simulink model "graphical_function4_2018a"  (R2018a)
settings: Solver=FixedStepDiscrete  StartTime=0.0  StopTime=1  FixedStep=0.1  RelTol=1e-3  EnableMultiTasking=on
settings Model: Creator=bzhan  LastModifiedBy=86188
settings SolverCC: AutoInsertRateTranBlk=on
settings DataIOCC: LimitDataPoints=on  ReturnWorkspaceOutputs=on
settings OptimizationCC: LifeSpan=inf
settings DebuggingCC: AllowSymbolicDim=off  SFUnexpectedBacktrackingDiag=warning  SFNoUnconditionalDefaultTransitionDiag=warning  SFExecutionAtInitializationDiag=none
settings CodeAppCC: StateflowObjectComments=on
settings GRTTargetCC: TargetLangStandard=C89/C90 (ANSI)
settings ConfigComp: CovMetricSettings=dw  CovHtmlReporting=on  CovSaveCumulativeToWorkspaceVar=on  CovSaveSingleToWorkspaceVar=on  CovShowResultsExplorer=off  CovExternalEMLEnable=off  CovSFcnEnable=off

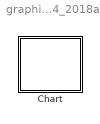
== system graphical_function4_2018a ==
  Chart : Stateflow chart  TreatAsAtomicUnit=on

== stateflow chart graphical_function4_2018a/Chart ==
  state flag=acked_all [function]
    (junction 40) -> (junction 49) [order 3]
    (junction 49) -> (junction 47) : {flag=0}
    (default) -> (junction 40) : {i=1}
    (junction 40) -> (junction 50) [order 1] : [i>2]
    (junction 50) -> (junction 47) : {flag=1}
    (junction 47) -> (junction 45)
    (junction 54) -> (junction 40)
    (junction 40) -> (junction 55) [order 2] : [i<=2]
    (junction 55) -> (junction 54) : {i = i + 1}
  state flag=empty [function]
    (junction 61) -> (junction 60) [order 3]
    (junction 60) -> (junction 63) : {flag=0}
    (default) -> (junction 61) : {i=first_SN}
    (junction 61) -> (junction 62) [order 1] : [i>last_SN]
    (junction 62) -> (junction 63) : {flag=1}
    (junction 63) -> (junction 64)
    (junction 65) -> (junction 61)
    (junction 61) -> (junction 66) [order 2] : [i<=last_SN&&unsent(i)==0]
    (junction 66) -> (junction 65) : {i = i + 1}
  state B
    en: f("en_B")
  state A
    en: f("en_A")
  (default) -> A
  A -> B : [acked_all()==true1&&empty()==false1]
  data: flag function_output; flag function_output; s function_input; last_SN local =5; first_SN local =1; unsent local size=[1 5] =[0 0 0 1 0]; false1 local =0; true1 local =1
  function f(s):
    | function f(s)
    |   fprintf(s+"\n");
